simulink model "PendulumHarnesses"  (R2025a)
settings: Solver=ode1be  StartTime=0.0  StopTime=6  FixedStep=0.001  RelTol=1e-3
settings Model: Creator=armte  LastModifiedBy=Глеб
settings OptimizationCC: ReuseModelBlockBuffer=off
settings RTWCC: GPUComputeCapability=3.5

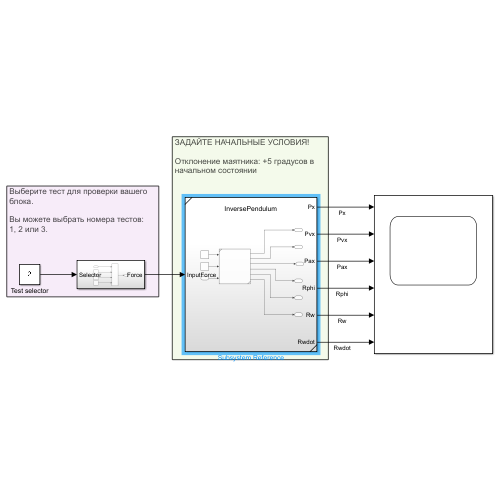
[thumbnail: Simulink's stored preview of the top-level diagram]
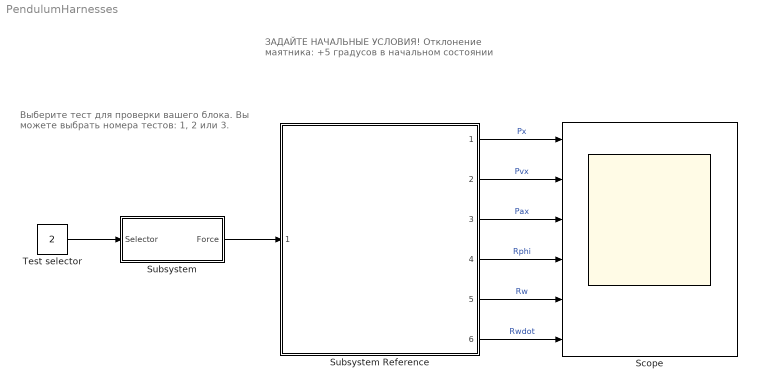
== system PendulumHarnesses ==
  note: ЗАДАЙТЕ НАЧАЛЬНЫЕ УСЛОВИЯ!
      |
      | Отклонение маятника: +5 градусов в
      | начальном состоянии
  note: Выберите тест для проверки вашего
      | блока.
      |
      | Вы можете выбрать номера тестов:
      | 1, 2 или 3.
  Scope : Scope  NumInputPorts=6
      settings: ActiveDisplayYMinimum=-1.7559935495154083E-14  ActiveDisplayYMaximum=1.9511039439060087E-15
  Subsystem : Subsystem
  Subsystem Reference : Subsystem  ReferencedSubsystem=InversePendulum
  Test selector : Constant  Value=2
  wires:
  Subsystem Reference/1 -> Scope/1  "Px"
  Subsystem Reference/2 -> Scope/2  "Pvx"
  Subsystem Reference/3 -> Scope/3  "Pax"
  Subsystem Reference/4 -> Scope/4  "Rphi"
  Subsystem Reference/5 -> Scope/5  "Rw"
  Subsystem Reference/6 -> Scope/6  "Rwdot"
  Test selector/1 -> Subsystem/1(Selector)
  Subsystem/1(Force) -> Subsystem Reference/1

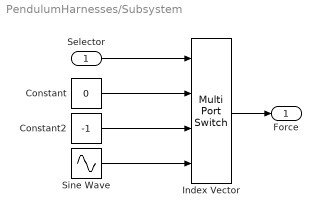
== system PendulumHarnesses/Subsystem ==
  Selector : Inport
  Constant : Constant  Value=0
  Constant2 : Constant  Value=-1
  Index Vector : MultiPortSwitch  SaturateOnIntegerOverflow=off  InputSameDT=off
  Sine Wave : Sin  Frequency=10  SampleTime=0
  Force : Outport
  wires:
  Index Vector/1 -> Force/1
  Selector/1 -> Index Vector/1
  Constant/1 -> Index Vector/2
  Constant2/1 -> Index Vector/3
  Sine Wave/1 -> Index Vector/4
